simulink model "M2"  (Simulink 7.3)
settings: Solver=ode5  StartTime=0.0  StopTime=10.0  FixedStep=0.02  RelTol=1e-3
undefined symbols (not defined in the file or in its folder): A, B, C, D, F1, F2, x0
settings Model: Creator=m134506  LastModifiedBy=m134506
settings DataIOCC: LimitDataPoints=off  TimeSaveName=t  OutputSaveName=run1

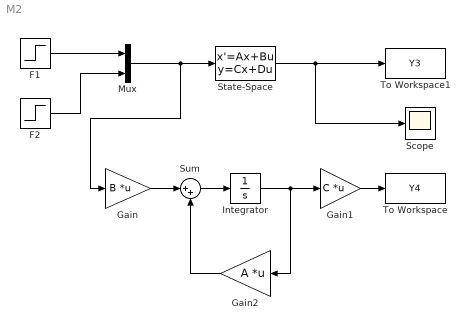
== system M2 ==
  F1 : Step  Time=0  After=F1  SampleTime=0
  F2 : Step  Time=0  After=F2  SampleTime=0
  Gain : Gain  Gain=B  Multiplication=Matrix(K*u)  ParameterDataType=fixdt(1, 16)  ParameterScaling=2^0  OutDataType=fixdt(1, 16)  OutScaling=2^0
  Gain1 : Gain  Gain=C  Multiplication=Matrix(K*u)  ParameterDataType=fixdt(1, 16)  ParameterScaling=2^0  OutDataType=fixdt(1, 16)  OutScaling=2^0
  Gain2 : Gain  Gain=A  Multiplication=Matrix(K*u)  ParameterDataType=fixdt(1, 16)  ParameterScaling=2^0  OutDataType=fixdt(1, 16)  OutScaling=2^0
  Integrator : Integrator  InitialCondition=x0
  Mux : Mux  Inputs=2
  Scope : Scope
  State-Space : StateSpace  A=A  B=B  C=C  D=D  X0=x0
  Sum : Sum  Inputs=|++  OutDataType=fixdt(1, 16)  OutScaling=2^0
  To Workspace : ToWorkspace  VariableName=Y4  SampleTime=-1  SaveFormat=Array
  To Workspace1 : ToWorkspace  VariableName=Y3  SampleTime=-1  SaveFormat=Array
  wires:
  Gain/1 -> Sum/1
  Gain2/1 -> Sum/2
  Sum/1 -> Integrator/1
  Integrator/1 -> Gain1/1, Gain2/1
  Gain1/1 -> To Workspace/1
  F1/1 -> Mux/1
  F2/1 -> Mux/2
  Mux/1 -> State-Space/1, Gain/1
  State-Space/1 -> To Workspace1/1, Scope/1
